simulink model "walden_prj_2_5_task3"  (R2025b)
settings: Solver=VariableStepAuto  StartTime=0.0  StopTime=10.0  RelTol=1e-3
libraries: slpidlib x1
settings Model: Creator=nrwal  LastModifiedBy=nrwal

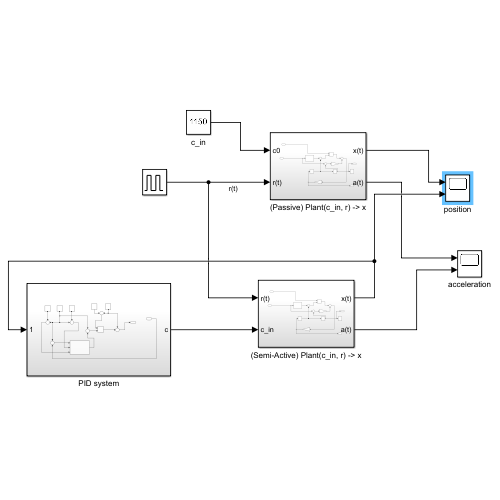
[thumbnail: Simulink's stored preview of the top-level diagram]
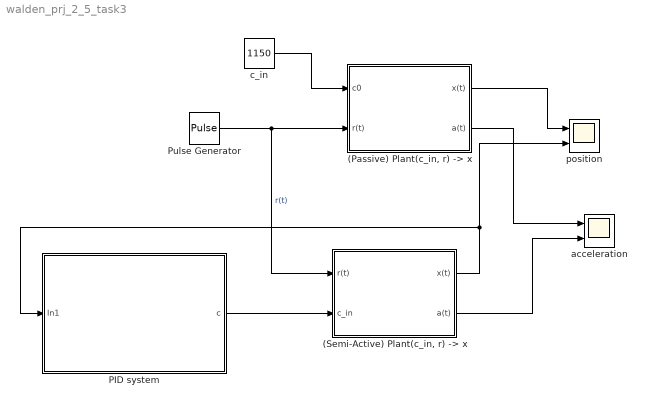
== system walden_prj_2_5_task3 ==
  "(Passive) Plant(c_in, r) -> x" : Subsystem
  "(Semi-Active) Plant(c_in, r) -> x" : Subsystem
  PID system : Subsystem
  Pulse Generator : DiscretePulseGenerator  PulseType=Time based  Amplitude=0.5  Period=10
  acceleration : Scope  NumInputPorts=2
      settings: ActiveDisplayYMinimum=-166.22989507394192  ActiveDisplayYMaximum=209.194454649382
  c_in : Constant  Value=1150
  position : Scope  NumInputPorts=2
      settings: ActiveDisplayYMinimum=-0.2280193743367859  ActiveDisplayYMaximum=0.36892350204718177
  wires:
  c_in/1 -> "(Passive) Plant(c_in, r) -> x"/1(c0)
  Pulse Generator/1 -> "(Semi-Active) Plant(c_in, r) -> x"/1(r(t)), "(Passive) Plant(c_in, r) -> x"/2(r(t))  "r(t)"
  "(Passive) Plant(c_in, r) -> x"/1(x(t)) -> position/1
  "(Semi-Active) Plant(c_in, r) -> x"/1(x(t)) -> PID system/1(In1), position/2
  PID system/1(c) -> "(Semi-Active) Plant(c_in, r) -> x"/2(c_in)
  "(Passive) Plant(c_in, r) -> x"/2(a(t)) -> acceleration/1
  "(Semi-Active) Plant(c_in, r) -> x"/2(a(t)) -> acceleration/2

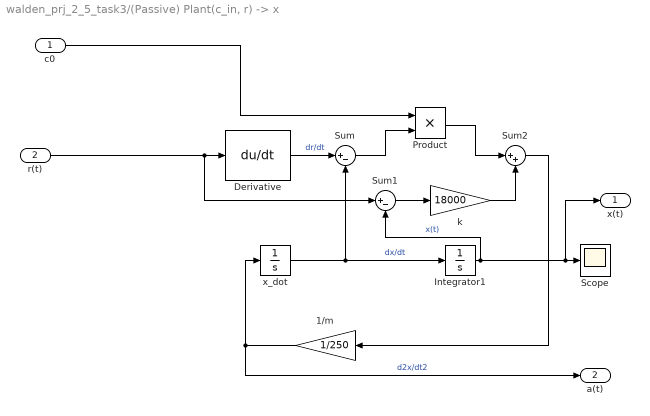
== system walden_prj_2_5_task3/(Passive) Plant(c_in, r) -> x ==
  c0 : Inport
  r(t) : Inport  Port=2
  1/m : Gain  Gain=1/250
  Derivative : Derivative
  Integrator1 : Integrator
  Product : Product
  Scope : Scope
      settings: ActiveDisplayYMinimum=-0.022050663065569576  ActiveDisplayYMaximum=0.021882842453229665
  Sum : Sum  Inputs=|+-
  Sum1 : Sum  Inputs=|+-
  Sum2 : Sum  Inputs=|++
  k : Gain  Gain=18000
  x_dot : Integrator
  x(t) : Outport
  a(t) : Outport  Port=2
  wires:
  1/m/1 -> a(t)/1, x_dot/1  "d2x/dt2"
  r(t)/1 -> Sum1/1, Derivative/1
  Derivative/1 -> Sum/1  "dr/dt"
  Sum1/1 -> k/1
  x_dot/1 -> Sum/2, Integrator1/1  "dx/dt"
  k/1 -> Sum2/2
  Product/1 -> Sum2/1
  Integrator1/1 -> Sum1/2, x(t)/1, Scope/1  "x(t)"
  Sum2/1 -> 1/m/1
  Sum/1 -> Product/2
  c0/1 -> Product/1

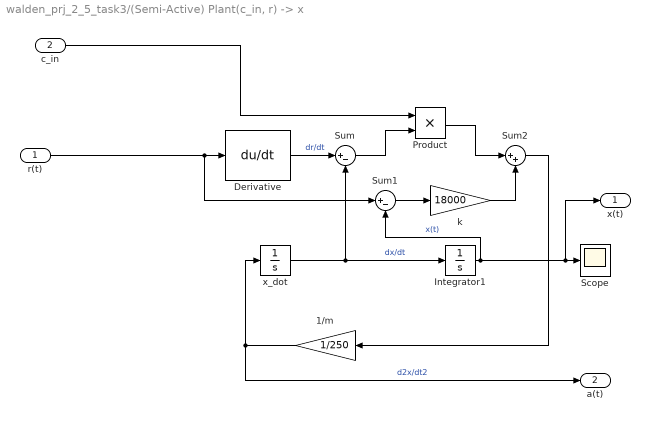
== system walden_prj_2_5_task3/(Semi-Active) Plant(c_in, r) -> x ==
  r(t) : Inport
  c_in : Inport  Port=2
  1/m : Gain  Gain=1/250
  Derivative : Derivative
  Integrator1 : Integrator
  Product : Product
  Scope : Scope
      settings: ActiveDisplayYMinimum=-0.022050663065569576  ActiveDisplayYMaximum=0.021882842453229665
  Sum : Sum  Inputs=|+-
  Sum1 : Sum  Inputs=|+-
  Sum2 : Sum  Inputs=|++
  k : Gain  Gain=18000
  x_dot : Integrator
  x(t) : Outport
  a(t) : Outport  Port=2
  wires:
  1/m/1 -> x_dot/1, a(t)/1  "d2x/dt2"
  r(t)/1 -> Sum1/1, Derivative/1
  Derivative/1 -> Sum/1  "dr/dt"
  Sum1/1 -> k/1
  x_dot/1 -> Sum/2, Integrator1/1  "dx/dt"
  k/1 -> Sum2/2
  Product/1 -> Sum2/1
  Integrator1/1 -> Sum1/2, x(t)/1, Scope/1  "x(t)"
  Sum2/1 -> 1/m/1
  Sum/1 -> Product/2
  c_in/1 -> Product/1

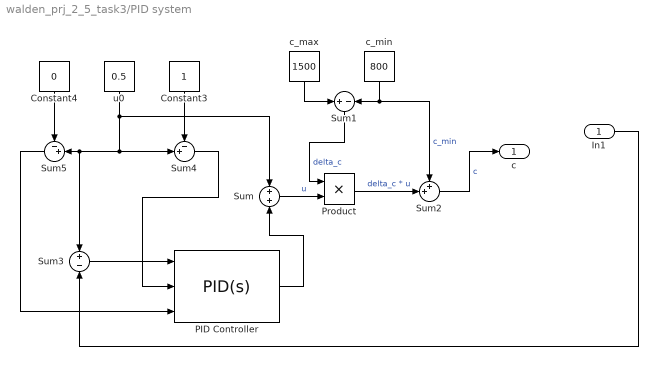
== system walden_prj_2_5_task3/PID system ==
  In1 : Inport
  Constant3 : Constant
  Constant4 : Constant  Value=0
  PID Controller : slpidlib/PID Controller  Controller=PID  Form=Parallel  TimeDomain=Continuous-time  UseExternalTs=off  SampleTime=-1  IntegratorMethod=Forward Euler  FilterMethod=Forward Euler  ControllerParametersSource=internal  P=200  I=500  UseKiTs=off  D=1  UseExternalDerivativeSource=off  N=100  UseFilter=on  TunerSelectOption=Transfer Function Based (PID Tuner App)  InitialConditionSource=internal  InitialConditionForIntegrator=0  InitialConditionForFilter=0  DifferentiatorICPrevScaledInput=0  ExternalReset=none  TrackingMode=off  Kt=1  LimitOutput=on  SatLimitsSource=external  UpperSaturationLimit=1  LowerSaturationLimit=0  LinearizeAsGain=on  AntiWindupMode=back-calculation  Kb=1  LimitIntegrator=on  UpperIntegratorSaturationLimit=inf  LowerIntegratorSaturationLimit=-inf  POutMin=[]  POutMax=[]  IOutMin=[]  IOutMax=[]  DOutMin=[]  DOutMax=[]  NOutMin=[]  NOutMax=[]  SumOutMin=[]  SumOutMax=[]  SaturationOutMin=[]  SaturationOutMax=[]  PParamMin=[]  PParamMax=[]  IParamMin=[]  IParamMax=[]  DParamMin=[]  DParamMax=[]  NParamMin=[]  NParamMax=[]  KbParamMin=[]  KbParamMax=[]  KtParamMin=[]  KtParamMax=[]  KbOutMin=[]  KbOutMax=[]  KtOutMin=[]  KtOutMax=[]  IntegratorOutMin=[]  IntegratorOutMax=[]  FilterOutMin=[]  FilterOutMax=[]  SumI1OutMin=[]  SumI1OutMax=[]  SumI2OutMin=[]  SumI2OutMax=[]  SumI3OutMin=[]  SumI3OutMax=[]  SumI4OutMin=[]  SumI4OutMax=[]  SumDOutMin=[]  SumDOutMax=[]  DifferentiatorOutMin=[]  DifferentiatorOutMax=[]  FilterDiffOutCoefMin=[]  FilterDiffOutCoefMax=[]  ReciprocalOutMin=[]  ReciprocalOutMax=[]  SumDenOutMin=[]  SumDenOutMax=[]  SumNumOutMin=[]  SumNumOutMax=[]  DivideOutMin=[]  DivideOutMax=[]  UdiffTsProdOutMin=[]  UdiffTsProdOutMax=[]  NTsProdOutMin=[]  NTsProdOutMax=[]  UintegralTsProdOutMin=[]  UintegralTsProdOutMax=[]  UngainTsProdOutMin=[]  UngainTsProdOutMax=[]  ClampingZeroOutDataTypeStr=Inherit: Inherit via back propagation  ClampingZeroOutMin=[]  ClampingZeroOutMax=[]  FilterDenConstantOutDataTypeStr=Inherit: Inherit via back propagation  FilterDenConstantOutMin=[]  FilterDenConstantOutMax=[]  PCopyOutDataTypeStr=Inherit: Inherit via back propagation  PCopyOutMin=[]  PCopyOutMax=[]  NCopyOutDataTypeStr=Inherit: Inherit via back propagation  NCopyOutMin=[]  NCopyOutMax=[]  IntegratorContinuousStateAttributes=''  IntegratorStateMustResolveToSignalObject=off  IntegratorRTWStateStorageClass=Auto  FilterContinuousStateAttributes=''  FilterStateMustResolveToSignalObject=off  FilterRTWStateStorageClass=Auto  ParallelPVariant=InternalParameters  IdealPVariant=Disabled  IVariant=InternalParameters  DVariant=InternalParameters  IntegratorVariant=Continuous  SatVariant=External  AWVariant=BackCalculation  PCopyVariant=Disabled  TRVariant=Disabled  FdbkBlocksVariant=Forward  IdealPFdbkVariant=Disabled  SatFdbkVariant=Disabled  DerivativeFilterVariant=ContFilter  NVariant=InternalParameters  NCopyVariant=Disabled  FilterICVariant=InternalICsFilter  IntegratorICVariant=InternalICs  ExternalResetVariant=Disabled  TRSumVariant=Passthrough  SumFdbkVariant=Disabled  SumVariant=Sum_PID  TsampFilterVariant=InternalTs  TsampNgainVariant=Passthrough  TsampIntegralVariant=Disabled_SignalSpec  ExternalSaturationOutDataTypeStr=Inherit: Same as second input  DerivativeSourceVariant=ErrorSignal  PreIntVariant=InternalPreInt
  Product : Product
  Sum : Sum
  Sum1 : Sum  Inputs=+|-
  Sum2 : Sum  Inputs=++|
  Sum3 : Sum  Inputs=+|-
  Sum4 : Sum  Inputs=-+|
  Sum5 : Sum  Inputs=-+|
  c_max : Constant  Value=1500
  c_min : Constant  Value=800
  u0 : Constant  Value=0.5
  c : Outport
  wires:
  Sum/1 -> Product/2  "u"
  Sum1/1 -> Product/1  "delta_c"
  c_min/1 -> Sum1/2, Sum2/1  "c_min"
  Constant3/1 -> Sum4/1
  Product/1 -> Sum2/2  "delta_c * u"
  u0/1 -> Sum/1, Sum5/2, Sum3/1, Sum4/2
  c_max/1 -> Sum1/1
  Sum3/1 -> PID Controller/1
  Sum5/1 -> PID Controller/3
  Constant4/1 -> Sum5/1
  Sum4/1 -> PID Controller/2
  PID Controller/1 -> Sum/2
  Sum2/1 -> c/1  "c"
  In1/1 -> Sum3/2
